simulink model "ACCModel"  (R2017b)
settings: Solver=VariableStepAuto  StartTime=0.0  StopTime=1  FixedStep=1  RelTol=1e-3
values from neighbouring files (symbols this model uses):
  dRelative = leadPoses.Position(1)    [DrivingSimulation.m]
  driverVel = 20    [DrivingSimulation.m]
  dSafe = 10    [ACCBreach.m]    (also in DrivingSimulation.m = 14.7)
  egoVel = egoMaxVel    (= 40)    [DrivingSimulation.m]
  K_rv = 5    [ACCBreach.m]    (also in DrivingSimulation.m)
  K_v = -1    [ACCBreach.m]    (also in DrivingSimulation.m)
  K_x = 1    [ACCBreach.m]    (also in DrivingSimulation.m)
settings Model: Creator=aniruddhgp  LastModifiedBy=puranic
settings CodeAppCC: StateflowObjectComments=on

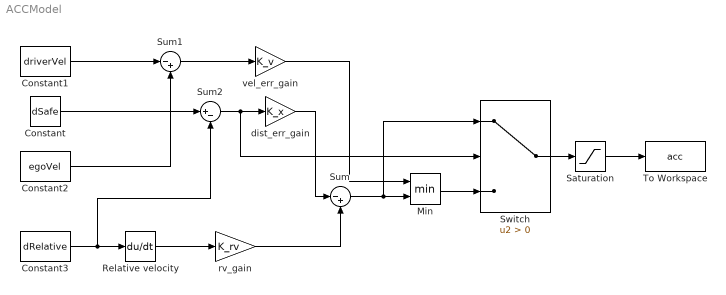
== system ACCModel ==
  Constant : Constant  Value=dSafe
  Constant1 : Constant  Value=driverVel
  Constant2 : Constant  Value=egoVel
  Constant3 : Constant  Value=dRelative
  Min : MinMax  Inputs=2
  Relative velocity : Derivative
  Saturation : Saturate  UpperLimit=3  LowerLimit=-inf
  Sum : Sum  Inputs=|-+
  Sum1 : Sum  Inputs=|-+
  Sum2 : Sum  Inputs=|+-
  Switch : Switch  Criteria=u2 > Threshold
  To Workspace : ToWorkspace  VariableName=acc  SaveFormat=Timeseries  SampleTime=-1
  dist_err_gain : Gain  Gain=K_x
  rv_gain : Gain  Gain=K_rv
  vel_err_gain : Gain  Gain=K_v
  wires:
  Relative velocity/1 -> rv_gain/1
  Switch/1 -> Saturation/1
  vel_err_gain/1 -> Min/1
  Sum2/1 -> Switch/2, dist_err_gain/1
  Min/1 -> Switch/3
  dist_err_gain/1 -> Sum/1
  Constant2/1 -> Sum1/2
  Sum1/1 -> vel_err_gain/1
  Constant/1 -> Sum2/1
  Sum/1 -> Switch/1, Min/2
  rv_gain/1 -> Sum/2
  Constant3/1 -> Sum2/2, Relative velocity/1
  Constant1/1 -> Sum1/1
  Saturation/1 -> To Workspace/1
